simulink model "w2_prob4_model"  (R2020a)
settings: Solver=ode15s  StartTime=0.0  StopTime=0.2  RelTol=1e-3
values from neighbouring files (symbols this model uses):
  B = 3.5077E-6    [w2_q4_214869.sldd]
  J = 3.2284E-6    [w2_q4_214869.sldd]
  K = 0.0274    [w2_q4_214869.sldd]
  L = 2.75E-6    [w2_q4_214869.sldd]
  R = 4.0    [w2_q4_214869.sldd]
undefined symbols (not defined in the file or in its folder): D, I, N, P
settings Model: DataDictionary=w2_q4_214869.sldd  Creator=sonal  LastModifiedBy=sonal
settings DataIOCC: SaveOutput=off  SaveTime=off

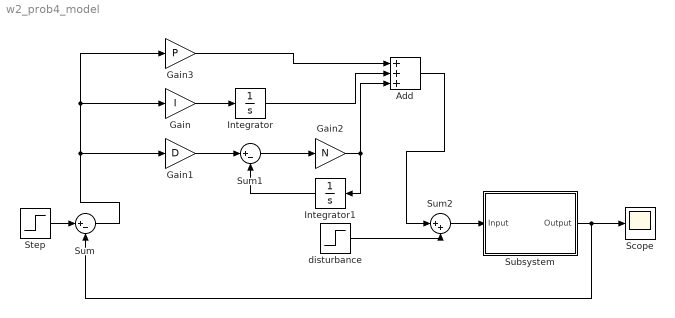
== system w2_prob4_model ==
  Add : Sum  Inputs=+++
  Gain : Gain  Gain=I
  Gain1 : Gain  Gain=D
  Gain2 : Gain  Gain=N
  Gain3 : Gain  Gain=P
  Integrator : Integrator
  Integrator1 : Integrator
  Scope : Scope
  Step : Step  Time=0  SampleTime=0
  Subsystem : Subsystem
  Sum : Sum  Inputs=|+-
  Sum1 : Sum  Inputs=|+-
  Sum2 : Sum  Inputs=|++
  disturbance : Step  Time=0.03  SampleTime=0
  wires:
  Step/1 -> Sum/1
  disturbance/1 -> Sum2/2
  Gain2/1 -> Add/3, Integrator1/1
  Sum1/1 -> Gain2/1
  Subsystem/1(Output) -> Sum/2, Scope/1
  Integrator1/1 -> Sum1/2
  Integrator/1 -> Add/2
  Gain3/1 -> Add/1
  Sum/1 -> Gain3/1, Gain/1, Gain1/1
  Gain/1 -> Integrator/1
  Gain1/1 -> Sum1/1
  Sum2/1 -> Subsystem/1(Input)
  Add/1 -> Sum2/1

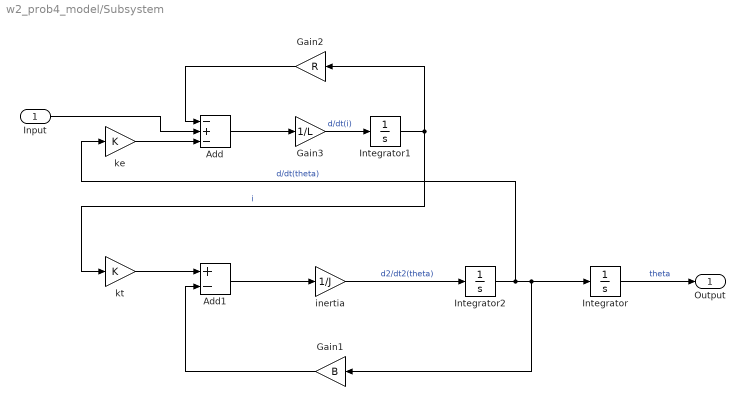
== system w2_prob4_model/Subsystem ==
  Input : Inport
  Add : Sum  Inputs=-+-
  Add1 : Sum  Inputs=+-
  Gain1 : Gain  Gain=B
  Gain2 : Gain  Gain=R
  Gain3 : Gain  Gain=1/L
  Integrator : Integrator
  Integrator1 : Integrator
  Integrator2 : Integrator
  inertia : Gain  Gain=1/J
  ke : Gain  Gain=K
  kt : Gain  Gain=K
  Output : Outport
  wires:
  Add1/1 -> inertia/1
  inertia/1 -> Integrator2/1  "d2/dt2(theta)"
  Integrator1/1 -> kt/1, Gain2/1  "i"
  Gain1/1 -> Add1/2
  Integrator/1 -> Output/1  "theta"
  Input/1 -> Add/2
  ke/1 -> Add/3
  Add/1 -> Gain3/1
  Gain3/1 -> Integrator1/1  "d/dt(i)"
  kt/1 -> Add1/1
  Integrator2/1 -> Integrator/1, Gain1/1, ke/1  "d/dt(theta)"
  Gain2/1 -> Add/1
